simulink model "control"  (Simulink 8.9)
settings: Solver=FixedStepAuto  StartTime=0.0  StopTime=3  MaxStep=0.01  RelTol=1e-4  EnableMultiTasking=on
libraries: fuzblock x1
settings Model: LogicAnalyzerSignalOrdering=33d7c2ba-298a-487f-a15a-bbe0029d2366,768ba1eb-50de-46f7-9be9-bebabd7bf970,4ab0f0e9-8454-41f6-a2d7-33861cd3e8d9  SuppressorTable=22 serialization::archive 11 0 6 0 0 0 11 0  Creator=root  LastModifiedBy=root
settings Model: LogicAnalyzerGraphicalSettings=|
  | {
  |   "cursors" : {
  |     "activeCursor" : 1,
  |     "lockedCursors" : [
  | 
  |     ],
  |     "startingCursor" : 0,
  |     "times" : [
  |       0,
  |       1.5341296928327646
  |     ]
  |   },
  |   "global" : {
  |   },
  |   "panels" : [
  |     {
  |       "height" : 100,
  |       "startingTrace" : 0,
  |       "traces" : [
  |         {
  |           "signalId" : "33d7c2ba-298a-487f-a15a-bbe0029d2366",
  |           "type" : "wave"
  |         },
  |         {
  |           "signalId" : "768ba1eb-50de-46f7-9be9-bebabd7bf970",
  |           "type" : "wave"
  |         },
  |         {
  |           "signalId" : "4ab0f0e9-8454-41f6-a2d7-33861cd3e8d9",
  |           "type" : "wave"
  |         }
  |       ],
  |       "yOffset" : 0
  |     }
  |   ],
  |   "timeAxis" : {
  |     "displayUnits" : "",
  |     "pixelsPerSecond" : 293
  |   }
  | }
settings DataIOCC: SaveFormat=Dataset  SignalLoggingSaveFormat=Dataset  SaveOutput=off  SaveTime=off
settings OptimizationCC: ExpressionDepthLimit=2147483647  LifeSpan=1
settings DebuggingCC: AllowSymbolicDim=off
settings HardwareCC: ProdBitPerPointer=64  ProdBitPerSizeT=64  ProdBitPerPtrDiffT=64  ProdLargestAtomicFloat=Float  ProdIntDivRoundTo=Zero  ProdEndianess=LittleEndian  ProdWordSize=64  ProdHWDeviceType=Intel->x86-64 (Windows64)
settings ModelReferenceCC: PropagateSignalLabelsOutOfModel=on
settings ConfigComp: CovMetricSettings=dwe  CovHtmlReporting=off  CovSaveCumulativeToWorkspaceVar=off  CovSaveSingleToWorkspaceVar=off  CovExternalEMLEnable=on

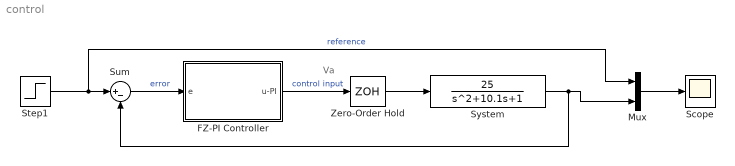
== system control ==
  note: Va
  FZ-PI Controller : Subsystem
  Mux : Mux  Inputs=2
  Scope : Scope
  Step1 : Step  Time=0  After=50  SampleTime=0
  Sum : Sum  Inputs=|+-
  System : TransferFcn  Numerator=[25]  Denominator=[1 10.1 1]
  Zero-Order Hold : ZeroOrderHold  SampleTime=0.01
  wires:
  Step1/1 -> Mux/1, Sum/1  "reference"
  Sum/1 -> FZ-PI Controller/1(e)  "error"
  FZ-PI Controller/1(u-PI) -> Zero-Order Hold/1  "control input"
  Zero-Order Hold/1 -> System/1
  System/1 -> Sum/2, Mux/2
  Mux/1 -> Scope/1

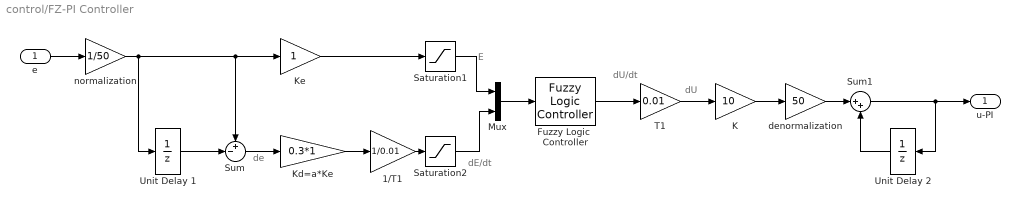
== system control/FZ-PI Controller ==
  note: E
  note: de
  note: dE/dt
  note: dU/dt
  note: dU
  e : Inport
  1/T1 : Gain  Gain=1/0.01
  "Fuzzy Logic  Controller " : fuzblock/Fuzzy Logic  Controller  fis='fis.fis'
  K : Gain  Gain=10
  Kd=a*Ke : Gain  Gain=0.3*1
  Mux : Mux  Inputs=2
  Saturation1 : Saturate  UpperLimit=1  LowerLimit=-1
  Saturation2 : Saturate  UpperLimit=1  LowerLimit=-1
  Sum : Sum  Inputs=+-|
  Sum1 : Sum  Inputs=|++
  "T1 " : Gain  Gain=0.01
  Unit Delay 1 : UnitDelay  SampleTime=0.01
  Unit Delay 2 : UnitDelay  SampleTime=0.01
  denormalization : Gain  Gain=50
  normalization : Gain  Gain=1/50
  Κe : Gain
  u-PI : Outport
  wires:
  e/1 -> normalization/1
  normalization/1 -> Unit Delay 1/1, Sum/1, Κe/1
  Unit Delay 1/1 -> Sum/2
  Sum/1 -> Kd=a*Ke/1
  Kd=a*Ke/1 -> 1/T1/1
  Κe/1 -> Saturation1/1
  1/T1/1 -> Saturation2/1
  Saturation1/1 -> Mux/1
  Saturation2/1 -> Mux/2
  "T1 "/1 -> K/1
  K/1 -> denormalization/1
  denormalization/1 -> Sum1/1
  Sum1/1 -> u-PI/1, Unit Delay 2/1
  Unit Delay 2/1 -> Sum1/2
  "Fuzzy Logic  Controller "/1 -> "T1 "/1
  Mux/1 -> "Fuzzy Logic  Controller "/1
